simulink model "Lab1_3_sol"  (R2015b)
settings: Solver=ode45  StartTime=0.0  StopTime=10000/20e6  RelTol=1e-3
undefined symbols (not defined in the file): fdesignblkfcn, gcbh, xlfda_numerator
libraries: xbsIndex_r4 x16, dsparch4 x1
(part 2 of 2)

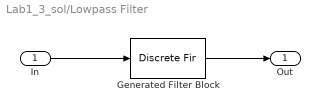
== system Lab1_3_sol/Lowpass Filter ==
  In : Inport
  Generated Filter Block : DiscreteFir  Tag=BlockMethodSubSystem  Coefficients=[0.006802019168867246 -0.0018271019166862348 -0.051845131678638426 0.0057350837125695478 0.29497742250115677 0.49199741364352395 0.29497742250115677 0.0057350837125695478 -0.051845131678638426 -0.0018271019166862348 0.006802019168867246]  InputProcessing=Columns as channels (frame based)
  Out : Outport
  wires:
  In/1 -> Generated Filter Block/1
  Generated Filter Block/1 -> Out/1
